simulink model "FOC_Motor_Control"  (R2020b)
settings: Solver=FixedStepAuto  StartTime=0.0  StopTime=10.0  FixedStep=Fixed_Step_Size  RelTol=1e-3
values from neighbouring files (symbols this model uses):
  Angle = 1.0    [Hall_FOC_Data.sldd]
  Angle_offset = 0.1985    [Hall_FOC_Data.sldd]
  atan_table = -1.5690511 -1.5690503 -1.5690495 -1.5690485 -1.5690477 -1.5690469 -1.569046 -1.5690452 -1.5690442 -1.5690434 -1.5690426 -1.5690417 -1.5690409 -1.5690399 -1.5690391 -1.5690383 -1.5690374 -1.5690365 -1.5690356 -1.5690348 -1.5690339 -1.569033 -1.5690322 -1.5690314 -1.5690304 -1.5690296 -1.5690287 -1.5690278 -1.5690269 -1.5690261 -1.5690252 -1.5690243 -1.5690234 -1.5690225 -1.5690217 -1.5690207 -1.569    [Hall_FOC_Data.sldd]
  Cosine_table = 1.0 0.99999529 0.99999058 0.99998587 0.99998116 0.99996704 0.99995291 0.99993885 0.99992472 0.99990118 0.99987763 0.99985409 0.9998306 0.99979764 0.99976468 0.99973178 0.99969882 0.99965644 0.99961412 0.99957174 0.99952942 0.99947762 0.99942589 0.99937415 0.99932235 0.9992612 0.99920005 0.99913889 0.99907768 0.99900717 0.99893659 0.99886602 0.99879545 0.99871546 0.99863547 0.99855554 0.99847555 0.    [Hall_FOC_Data.sldd]
  Dead_Com_Enable = 0.0    [Hall_FOC_Data.sldd]
  Dead_Time = 0.0    [Hall_FOC_Data.sldd]
  FF_Enable = 0.0    [Hall_FOC_Data.sldd]
  Flux = 0.0260812    [Hall_FOC_Data.sldd]
  FluxWeak_Enable = 0.0    [Hall_FOC_Data.sldd]
  FluxWeak_Idref_max = 0.0    [Hall_FOC_Data.sldd]
  FluxWeak_Idref_min = -200.0    [Hall_FOC_Data.sldd]
  FluxWeak_Ki = 50.0    [Hall_FOC_Data.sldd]
  FluxWeak_Kp = 1.2    [Hall_FOC_Data.sldd]
  HaLL_AngleShift = -0.25    [Hall_FOC_Data.sldd]
  HaLL_Sector1 = 5.236    [Hall_FOC_Data.sldd]
  HaLL_Sector2 = 1.0472    [Hall_FOC_Data.sldd]
  HaLL_Sector3 = 0.0    [Hall_FOC_Data.sldd]
  HaLL_Sector4 = 3.1415    [Hall_FOC_Data.sldd]
  HaLL_Sector5 = 4.1888    [Hall_FOC_Data.sldd]
  HaLL_Sector6 = 2.0944    [Hall_FOC_Data.sldd]
  HaLL_Timer_T = 1.0E-5    [Hall_FOC_Data.sldd]
  Harmonic_Com_Enable = 0.0    [Hall_FOC_Data.sldd]
  Harmonic_Id5th_Ki = 32.0    [Hall_FOC_Data.sldd]
  Harmonic_Id5th_Kp = 1.2    [Hall_FOC_Data.sldd]
  Harmonic_Id5th_Max = 60.0    [Hall_FOC_Data.sldd]
  Harmonic_Id5th_Min = -60.0    [Hall_FOC_Data.sldd]
  Harmonic_Id7th_Ki = 24.0    [Hall_FOC_Data.sldd]
  Harmonic_Id7th_Kp = 0.8    [Hall_FOC_Data.sldd]
  Harmonic_Id7th_Max = 60.0    [Hall_FOC_Data.sldd]
  Harmonic_Id7th_Min = -60.0    [Hall_FOC_Data.sldd]
  Harmonic_Iq5th_Ki = 32.0    [Hall_FOC_Data.sldd]
  Harmonic_Iq5th_Kp = 1.2    [Hall_FOC_Data.sldd]
  Harmonic_Iq5th_Max = 60.0    [Hall_FOC_Data.sldd]
  Harmonic_Iq5th_Min = -60.0    [Hall_FOC_Data.sldd]
  Harmonic_Iq7th_Ki = 24.0    [Hall_FOC_Data.sldd]
  Harmonic_Iq7th_Kp = 0.8    [Hall_FOC_Data.sldd]
  Harmonic_Iq7th_Max = 60.0    [Hall_FOC_Data.sldd]
  Harmonic_Iq7th_Min = -60.0    [Hall_FOC_Data.sldd]
  ID_Ki = 0.8    [Hall_FOC_Data.sldd]
  ID_Kp = 3.2    [Hall_FOC_Data.sldd]
  IQ_Ki = 0.32    [Hall_FOC_Data.sldd]
  IQ_Kp = 3.3    [Hall_FOC_Data.sldd]
  LADRC_b0 = 80000.0    [Hall_FOC_Data.sldd]
  LADRC_Omega_c = 80.0    [Hall_FOC_Data.sldd]
  Ld = 0.004    [Hall_FOC_Data.sldd]
  Lq = 0.0042    [Hall_FOC_Data.sldd]
  MTPA_id_table = 0.22889 0.23462678 0.23770036 0.2381243 0.23591207 0.23107713 0.2236329 0.21359272 0.20096992 0.18577772 0.16802935 0.14773798 0.12491672 0.099578641 0.071736768 0.041404068 0.0085934745 -0.026682133 -0.064409919 -0.10457709 -0.14717092 -0.1921787 -0.2395878 -0.28938559 -0.34155953 -0.39609709 -0.45298585 -0.51221335 -0.57376724 -0.63763517 -0.70380485 -0.77226412 -0.84300071 -0.91600245 -0.991257    [Hall_FOC_Data.sldd]
  MTPA_iq_table = -1.0417 -0.16083497 0.71926296 1.5985928 2.4771533 3.3549435 4.2319627 5.1082091 5.9836826 6.8583813 7.732305 8.6054525 9.4778223 10.349415 11.220228 12.090261 12.959513 13.827983 14.69567 15.562573 16.428694 17.294027 18.158575 19.022335 19.885307 20.747492 21.608887 22.469492 23.329306 24.188328 25.046556 25.903992 26.760633 27.616482 28.471533 29.325788 30.179247 31.031908 31.883772 32.734837 3    [Hall_FOC_Data.sldd]
  MTPA_Te_Max = 800.0    [Hall_FOC_Data.sldd]
  MTPA_Te_Min = 0.0    [Hall_FOC_Data.sldd]
  Over_modulation = 0.0    [Hall_FOC_Data.sldd]
  Pole_Pairs = 2.0    [Hall_FOC_Data.sldd]
  PWM_Frequency = 10000.0    [Hall_FOC_Data.sldd]
  R = 0.4    [Hall_FOC_Data.sldd]
  Sine_table = 0.0 0.0015339879 0.0030679768 0.0046019657 0.0061359555 0.0076698866 0.0092038177 0.010737749 0.012271681 0.013805497 0.015339312 0.016873131 0.018406944 0.019940587 0.021474229 0.023007872 0.024541514 0.026074925 0.027608337 0.029141748 0.03067516 0.032208283 0.033741407 0.035274528 0.036807653 0.038340431 0.039873205 0.04140598 0.042938754 0.04447113 0.046003502 0.047535874 0.049068246 0.0506001    [Hall_FOC_Data.sldd]
  Speed_Ki = 0.633    [Hall_FOC_Data.sldd]
  Speed_Kp = 0.0267    [Hall_FOC_Data.sldd]
  Speed_PI_OutputMax = 5.0    [Hall_FOC_Data.sldd]
  Speed_PI_OutputMin = -5.0    [Hall_FOC_Data.sldd]
  SpeedFilter_Fn = 0.2    [Hall_FOC_Data.sldd]
  TorqueMode = 0.0    [Hall_FOC_Data.sldd]
undefined symbols (not defined in the file or in its folder): DiscIntNeverNeededParam, inverter, magnitude, SVPWM
libraries: simulink x6, powerlib_extras x4, pid_lib x1
(part 4 of 5)

== system FOC_Motor_Control/Motor_Control/Motor_Control_Function/Angle_Speed_100us/SpeedAndAngle/ADC_IRQ/HallAngle_calibration/If Action Subsystem1 ==
  In1 : Inport
  Action Port : ActionPort  ActionPortLabel=else
  Out1 : Outport
  wires:
  In1/1 -> Out1/1

== system FOC_Motor_Control/Motor_Control/Motor_Control_Function/Angle_Speed_100us/SpeedAndAngle/ADC_IRQ/HallAngle_calibration/If Action Subsystem2 ==
  In1 : Inport
  Action Port : ActionPort  ActionPortLabel=if(u1 > 6.283185307)
  2pi : Constant  Value=2*pi  OutDataTypeStr=single
  Subtract1 : Sum  Inputs=+-  OutDataTypeStr=single
  Out1 : Outport
  wires:
  In1/1 -> Subtract1/1
  Subtract1/1 -> Out1/1
  2pi/1 -> Subtract1/2

== system FOC_Motor_Control/Motor_Control/Motor_Control_Function/Angle_Speed_100us/SpeedAndAngle/ADC_IRQ/HallAngle_calibration/If Action Subsystem3 ==
  In1 : Inport
  Action Port : ActionPort  ActionPortLabel=elseif(u1<0)
  Angle_offset : Constant  Value=2*pi  OutDataTypeStr=single
  Subtract1 : Sum
  Out1 : Outport
  wires:
  In1/1 -> Subtract1/1
  Subtract1/1 -> Out1/1
  Angle_offset/1 -> Subtract1/2

== system FOC_Motor_Control/Motor_Control/Motor_Control_Function/Control_Command_2ms/Control_Command_2ms/Speed_PI/SpeedLoop/LESO ==
  FbkSpd : Inport  OutDataTypeStr=single  PortDimensions=1
  iq : Inport  Port=2  OutDataTypeStr=single  PortDimensions=1
  Reset : Inport  Port=3
  Constant : Constant  Value=LADRC_Omega_c  OutDataTypeStr=single
  Constant1 : Constant  Value=LADRC_b0  OutDataTypeStr=single  SampleTime=-1
  Discrete-Time Integrator : DiscreteIntegrator  ExternalReset=level  SampleTime=-1  OutDataTypeStr=single  UpperSaturationLimit=6e4  LowerSaturationLimit=-6e4  ICPrevOutput=DiscIntNeverNeededParam  ICPrevScaledInput=DiscIntNeverNeededParam
  Discrete-Time Integrator1 : DiscreteIntegrator  ExternalReset=level  SampleTime=-1  OutDataTypeStr=single  LimitOutput=on  UpperSaturationLimit=2000  LowerSaturationLimit=-2000  ICPrevOutput=DiscIntNeverNeededParam  ICPrevScaledInput=DiscIntNeverNeededParam
  Gain : Gain  Gain=3  OutDataTypeStr=single
  Gain1 : Gain  Gain=2  OutDataTypeStr=single
  Product : Product  Inputs=3  OutDataTypeStr=single
  Product1 : Product  OutDataTypeStr=single
  Product2 : Product  OutDataTypeStr=single
  Sum : Sum  Inputs=|+-  OutDataTypeStr=single
  Sum1 : Sum  Inputs=+++  OutDataTypeStr=single
  omega_r_hat : Outport  OutDataTypeStr=single
  f_hat : Outport  Port=2  OutDataTypeStr=single
  wires:
  Sum/1 -> Gain1/1, Product/3
  Product/1 -> Discrete-Time Integrator/1
  Discrete-Time Integrator/1 -> [f_hat], f_hat/1
  [f_hat] -> Sum1/3
  Sum1/1 -> Discrete-Time Integrator1/1
  Discrete-Time Integrator1/1 -> omega_r_hat/1, [omega_r_hat]
  Product1/1 -> Sum1/1
  FbkSpd/1 -> Sum/1
  [omega_r_hat] -> Sum/2
  Constant/1 -> Gain/1
  Gain1/1 -> Product1/2
  Gain/1 -> Product1/1, Product/2, Product/1
  iq/1 -> Product2/1
  Constant1/1 -> Product2/2
  Product2/1 -> Sum1/2
  Reset/1 -> Discrete-Time Integrator/2, Discrete-Time Integrator1/2

== system FOC_Motor_Control/Motor_Control/Motor_Control_Function/Control_Command_2ms/Control_Command_2ms/Speed_PI/Speed_PI/Speed_Control ==
  Err : Inport
  Reset : Inport  Port=2
  Add : Sum
  Cons : Constant  Value=0  OutDataTypeStr=single
  Discrete-Time Integrator : DiscreteIntegrator  ExternalReset=level  SampleTime=-1  ICPrevOutput=DiscIntNeverNeededParam  ICPrevScaledInput=DiscIntNeverNeededParam
  Ki : Constant  Value=Speed_Ki  OutDataTypeStr=single
  Kp : Constant  Value=Speed_Kp  OutDataTypeStr=single
  Product : Product
  Product1 : Product
  Relational Operator1 : RelationalOperator  Operator===  OutDataTypeStr=boolean  RndMeth=Simplest
  Saturation : Saturate  UpperLimit=Speed_PI_OutputMax  LowerLimit=Speed_PI_OutputMin
  Scope : Scope
  Switch : Switch  Criteria=u2 > Threshold
  Unit Delay3 : UnitDelay  SampleTime=-1  HasFrameUpgradeWarning=on
  PI_Out : Outport
  wires:
  Kp/1 -> Product/1
  Err/1 -> Switch/1, Product/2
  Switch/1 -> Product1/2
  Product1/1 -> Discrete-Time Integrator/1
  Product/1 -> Add/1
  Add/1 -> Relational Operator1/1, Saturation/1
  Saturation/1 -> Relational Operator1/2, PI_Out/1
  Discrete-Time Integrator/1 -> Add/2, Scope/1
  Relational Operator1/1 -> Unit Delay3/1
  Ki/1 -> Product1/1
  Unit Delay3/1 -> Switch/2
  Cons/1 -> Switch/3
  Reset/1 -> Discrete-Time Integrator/2

== system FOC_Motor_Control/Motor_Control/Motor_Control_Function/Control_Command_2ms/Flux_weakening /Subsystem/Flux_weak/ID_Control ==
  Err : Inport
  Reset : Inport  Port=2
  Add : Sum
  Cons : Constant  Value=0  OutDataTypeStr=single
  Discrete-Time Integrator : DiscreteIntegrator  ExternalReset=level  SampleTime=-1  ICPrevOutput=DiscIntNeverNeededParam  ICPrevScaledInput=DiscIntNeverNeededParam
  Ki : Constant  Value=ki  OutDataTypeStr=single
  Kp : Constant  Value=kp  OutDataTypeStr=single
  Product : Product
  Product1 : Product
  Relational Operator1 : RelationalOperator  Operator===  OutDataTypeStr=boolean  RndMeth=Simplest
  Saturation : Saturate  UpperLimit=Id_max  LowerLimit=Id_min
  Switch : Switch  Criteria=u2 > Threshold
  Unit Delay3 : UnitDelay  SampleTime=-1  HasFrameUpgradeWarning=on
  PI_Out : Outport
  wires:
  Kp/1 -> Product/1
  Err/1 -> Switch/1, Product/2
  Switch/1 -> Product1/2
  Product1/1 -> Discrete-Time Integrator/1
  Product/1 -> Add/1
  Add/1 -> Relational Operator1/1, Saturation/1
  Saturation/1 -> Relational Operator1/2, PI_Out/1
  Cons/1 -> Switch/3
  Discrete-Time Integrator/1 -> Add/2
  Relational Operator1/1 -> Unit Delay3/1
  Ki/1 -> Product1/1
  Unit Delay3/1 -> Switch/2
  Reset/1 -> Discrete-Time Integrator/2

== system FOC_Motor_Control/Motor_Control/Motor_Control_Function/Control_Command_2ms/Flux_weakening /Subsystem/Flux_weak/Normal ==
  Bus_voltage : Inport
  Action Port : ActionPort  ActionPortLabel=elseif(u1==0)
  Gain : Gain  Gain=1/sqrt(3)
  Out1 : Outport
  wires:
  Bus_voltage/1 -> Gain/1
  Gain/1 -> Out1/1

== system FOC_Motor_Control/Motor_Control/Motor_Control_Function/Control_Command_2ms/Flux_weakening /Subsystem/Flux_weak/Over_M ==
  Bus_voltage : Inport
  Action Port : ActionPort  ActionPortLabel=if(u1==1)
  Gain : Gain  Gain=2/3
  Out1 : Outport
  wires:
  Bus_voltage/1 -> Gain/1
  Gain/1 -> Out1/1

== system FOC_Motor_Control/Motor_Control/Motor_Control_Function/FOC_Control_100us/FOC/DT_Compensation/DT_Compensation/IsTheta_Cal ==
  Id : Inport
  Iq : Inport  Port=2
  d_theta : Inport  Port=3
  Add1 : Sum
  Angle_calibration : Subsystem
      settings: RTWSystemCode=Nonreusable function  RTWFcnNameOpts=Use subsystem name
  LPF : Subsystem
  LPF1 : Subsystem
  Scope2 : Scope  NumInputPorts=2
  Scope3 : Scope  NumInputPorts=2
  atan : Subsystem
  IsTheta : Outport
  wires:
  d_theta/1 -> Add1/2
  Angle_calibration/1(Angle_output) -> IsTheta/1
  Iq/1 -> LPF/1(u), Scope2/1
  Id/1 -> LPF1/1(u), Scope3/1
  LPF1/1(y) -> [B_Id], Scope3/2
  LPF/1(y) -> Scope2/2, [A_Iq]
  Add1/1 -> Angle_calibration/1(Angle_input)  "Itheta2"
  [A_Iq] -> atan/1(Id)
  [B_Id] -> atan/2(Iq)
  atan/1(Out1) -> Add1/1

== system FOC_Motor_Control/Motor_Control/Motor_Control_Function/FOC_Control_100us/FOC/DT_Compensation/DT_Compensation/Subsystem ==
  Err_Voltage : Inport
  Istheta : Inport  Port=2
  If1 : If  IfExpression=(u1 >5.75958)|(u1<=0.523598)  ElseIfExpressions=(u1 >0.523598)&(u1<=1.570796),(u1 >1.570796)&(u1<=2.617993),(u1 >2.617993)&(u1<=3.665191),(u1 >3.665191)&(u1<=4.7123889),(u1 >4.7123889)&(u1<=5.75958)  ShowElse=off
  Merge : Merge  Inputs=6
  Subsystem : Subsystem
  Subsystem1 : Subsystem
  Subsystem2 : Subsystem
  Subsystem3 : Subsystem
  Subsystem4 : Subsystem
  Subsystem5 : Subsystem
  Uabcc : Outport
  wires:
  Istheta/1 -> If1/1
  If1/1 -> Subsystem/Action
  If1/2 -> Subsystem1/Action
  If1/3 -> Subsystem2/Action
  If1/4 -> Subsystem3/Action
  If1/5 -> Subsystem4/Action
  If1/6 -> Subsystem5/Action
  Err_Voltage/1 -> Subsystem5/1(Voltage), Subsystem3/1(Voltage), Subsystem2/1(Voltage), Subsystem/1(Voltage), Subsystem1/1(Voltage), Subsystem4/1(Voltage)
  Merge/1 -> Uabcc/1
  Subsystem/1(Out1) -> Merge/1
  Subsystem1/1(Out1) -> Merge/2
  Subsystem2/1(Out1) -> Merge/3
  Subsystem3/1(Out1) -> Merge/4
  Subsystem4/1(Out1) -> Merge/5
  Subsystem5/1(Out1) -> Merge/6

== system FOC_Motor_Control/Motor_Control/Motor_Control_Function/FOC_Control_100us/FOC/DT_Compensation/DT_Compensation/Uabc_alphabeta ==
  Uabc : Inport
  Fcn : Fcn  Expr=(2/3)*(u(1)-0.5*u(2)-0.5*u(3))
  Fcn1 : Fcn  Expr=sqrt(1/3)*(u(2)-u(3))
  Ualpha : Outport
  Ubeta : Outport  Port=2
  wires:
  Fcn/1 -> Ualpha/1
  Fcn1/1 -> Ubeta/1
  Uabc/1 -> Fcn1/1, Fcn/1

== system FOC_Motor_Control/Motor_Control/Motor_Control_Function/FOC_Control_100us/FOC/D_Current_PI/ID_Control/Normal ==
  Bus_voltage : Inport
  Action Port : ActionPort  ActionPortLabel=elseif(u1==0)
  Gain : Gain  Gain=1/sqrt(3)
  Gain1 : Gain  Gain=-1/sqrt(3)
  Out1 : Outport
  Out2 : Outport  Port=2
  wires:
  Bus_voltage/1 -> Gain1/1, Gain/1
  Gain/1 -> Out1/1
  Gain1/1 -> Out2/1

== system FOC_Motor_Control/Motor_Control/Motor_Control_Function/FOC_Control_100us/FOC/D_Current_PI/ID_Control/Over_M ==
  Bus_voltage : Inport
  Action Port : ActionPort  ActionPortLabel=if(u1==1)
  Gain : Gain  Gain=2/3
  Gain1 : Gain  Gain=-2/3
  Out1 : Outport
  Out2 : Outport  Port=2
  wires:
  Bus_voltage/1 -> Gain1/1, Gain/1
  Gain/1 -> Out1/1
  Gain1/1 -> Out2/1

== system FOC_Motor_Control/Motor_Control/Motor_Control_Function/FOC_Control_100us/FOC/Har_Compensation/Har_Compensation/Idq5 ==
  Ialpha : Inport
  Ibeta : Inport  Port=2
  Cos_theta : Inport  Port=3
  Sin_theta : Inport  Port=4
  LPF : Subsystem
  LPF2 : Subsystem
  Mux : Mux  Inputs=2
  Park1 : Subsystem
  Scope : Scope  NumInputPorts=2
  Idq5 : Outport  VectorParamsAs1DForOutWhenUnconnected=off
  wires:
  Park1/1(Id5) -> Mux/1
  Park1/2(Iq5) -> Mux/2
  Mux/1 -> Scope/1, LPF/1(u)
  Cos_theta/1 -> Park1/3(Cos_theta)
  Sin_theta/1 -> Park1/4(Sin_theta)
  Ialpha/1 -> Park1/1(Ialf)
  Ibeta/1 -> Park1/2(Ibelt)
  LPF/1(y) -> LPF2/1(u)
  LPF2/1(y) -> Scope/2, Idq5/1

== system FOC_Motor_Control/Motor_Control/Motor_Control_Function/FOC_Control_100us/FOC/Har_Compensation/Har_Compensation/Idq7 ==
  Ialpha : Inport
  Ibeta : Inport  Port=2
  Cos_theta : Inport  Port=3
  Sin_theta : Inport  Port=4
  LPF : Subsystem
  LPF2 : Subsystem
  Mux : Mux  Inputs=2
  Park1 : Subsystem
  Idq7 : Outport  VectorParamsAs1DForOutWhenUnconnected=off
  wires:
  Park1/2(Iq7) -> Mux/2
  Ibeta/1 -> Park1/2(Ibelt)
  Ialpha/1 -> Park1/1(Ialf)
  Park1/1(Id7) -> Mux/1
  Mux/1 -> LPF/1(u)
  Sin_theta/1 -> Park1/4(Sin_theta)
  Cos_theta/1 -> Park1/3(Cos_theta)
  LPF/1(y) -> LPF2/1(u)
  LPF2/1(y) -> Idq7/1

== system FOC_Motor_Control/Motor_Control/Motor_Control_Function/FOC_Control_100us/FOC/Har_Compensation/Har_Compensation/Sine_Cosine1 ==
  note: Sine Cosine Coefficients
  P : Inport
  Cosine : Lookup_n-D  NumberOfTableDimensions=1  LookupTableObject=''  BreakpointsForDimension1=[0:2*pi/4095:2*pi]  BreakpointsForDimension1FirstPoint=10  BreakpointsForDimension2FirstPoint=10  BreakpointsForDimension1Spacing=12  BreakpointsForDimension2Spacing=12  IndexSearchMethod=Evenly spaced points  Table=Cosine_table  InterpMethod=Flat  DiagnosticForOutOfRangeInput=Error  InternalRulePriority=Speed  RndMeth=Simplest  InputSameDT=on
  Saturation : Saturate  UpperLimit=2*pi-0.0001  LowerLimit=0+0.0001
  Scope : Scope  NumInputPorts=2
  Sine : Lookup_n-D  NumberOfTableDimensions=1  LookupTableObject=''  BreakpointsForDimension1=[0:2*pi/4095:2*pi]  BreakpointsForDimension1FirstPoint=10  BreakpointsForDimension2FirstPoint=10  BreakpointsForDimension1Spacing=12  BreakpointsForDimension2Spacing=12  IndexSearchMethod=Evenly spaced points  Table=Sine_table  InterpMethod=Flat  DiagnosticForOutOfRangeInput=Error  InternalRulePriority=Speed  RndMeth=Simplest  InputSameDT=on
  Cos : Outport  VectorParamsAs1DForOutWhenUnconnected=off
  Sin : Outport  Port=2  VectorParamsAs1DForOutWhenUnconnected=off
  wires:
  P/1 -> Saturation/1  "position"
  Sine/1 -> Scope/1, Sin/1
  Cosine/1 -> Scope/2, Cos/1
  Saturation/1 -> Cosine/1, Sine/1

== system FOC_Motor_Control/Motor_Control/Motor_Control_Function/FOC_Control_100us/FOC/Har_Compensation/Har_Compensation/Sine_Cosine2 ==
  note: Sine Cosine Coefficients
  P : Inport
  Cosine : Lookup_n-D  NumberOfTableDimensions=1  LookupTableObject=''  BreakpointsForDimension1=[0:2*pi/4095:2*pi]  BreakpointsForDimension1FirstPoint=10  BreakpointsForDimension2FirstPoint=10  BreakpointsForDimension1Spacing=12  BreakpointsForDimension2Spacing=12  IndexSearchMethod=Evenly spaced points  Table=Cosine_table  InterpMethod=Flat  DiagnosticForOutOfRangeInput=Error  InternalRulePriority=Speed  RndMeth=Simplest  InputSameDT=on
  Saturation : Saturate  UpperLimit=2*pi-0.0001  LowerLimit=0+0.0001
  Scope : Scope  NumInputPorts=2
  Sine : Lookup_n-D  NumberOfTableDimensions=1  LookupTableObject=''  BreakpointsForDimension1=[0:2*pi/4095:2*pi]  BreakpointsForDimension1FirstPoint=10  BreakpointsForDimension2FirstPoint=10  BreakpointsForDimension1Spacing=12  BreakpointsForDimension2Spacing=12  IndexSearchMethod=Evenly spaced points  Table=Sine_table  InterpMethod=Flat  DiagnosticForOutOfRangeInput=Error  InternalRulePriority=Speed  RndMeth=Simplest  InputSameDT=on
  Cos : Outport  VectorParamsAs1DForOutWhenUnconnected=off
  Sin : Outport  Port=2  VectorParamsAs1DForOutWhenUnconnected=off
  wires:
  P/1 -> Saturation/1  "position"
  Sine/1 -> Scope/1, Sin/1
  Cosine/1 -> Scope/2, Cos/1
  Saturation/1 -> Cosine/1, Sine/1

== system FOC_Motor_Control/Motor_Control/Motor_Control_Function/FOC_Control_100us/FOC/Har_Compensation/Har_Compensation/Switch_2pi ==
  Input : Inport
  Data Type Conversion : DataTypeConversion  OutDataTypeStr=int32
  Divide : Product  Inputs=*/
  Divide1 : Product  Inputs=**
  Subtract : Sum  Inputs=-+
  Te2 : Constant  Value=2*pi  OutDataTypeStr=single
  Te3 : Constant  Value=2*pi  OutDataTypeStr=single
  output : Outport
  wires:
  Te3/1 -> Divide1/2
  Data Type Conversion/1 -> Divide1/1
  Divide/1 -> Data Type Conversion/1
  Divide1/1 -> Subtract/1
  Te2/1 -> Divide/2
  Subtract/1 -> output/1
  Input/1 -> Subtract/2, Divide/1

== system FOC_Motor_Control/Motor_Control/Motor_Control_Function/FOC_Control_100us/FOC/Har_Compensation/Har_Compensation/Switch_2pi1 ==
  Input : Inport
  Data Type Conversion : DataTypeConversion  OutDataTypeStr=int32
  Divide : Product  Inputs=*/
  Divide1 : Product  Inputs=**
  Subtract : Sum  Inputs=-+
  Te2 : Constant  Value=2*pi  OutDataTypeStr=single
  Te3 : Constant  Value=2*pi  OutDataTypeStr=single
  output : Outport
  wires:
  Te3/1 -> Divide1/2
  Data Type Conversion/1 -> Divide1/1
  Divide/1 -> Data Type Conversion/1
  Divide1/1 -> Subtract/1
  Te2/1 -> Divide/2
  Subtract/1 -> output/1
  Input/1 -> Subtract/2, Divide/1

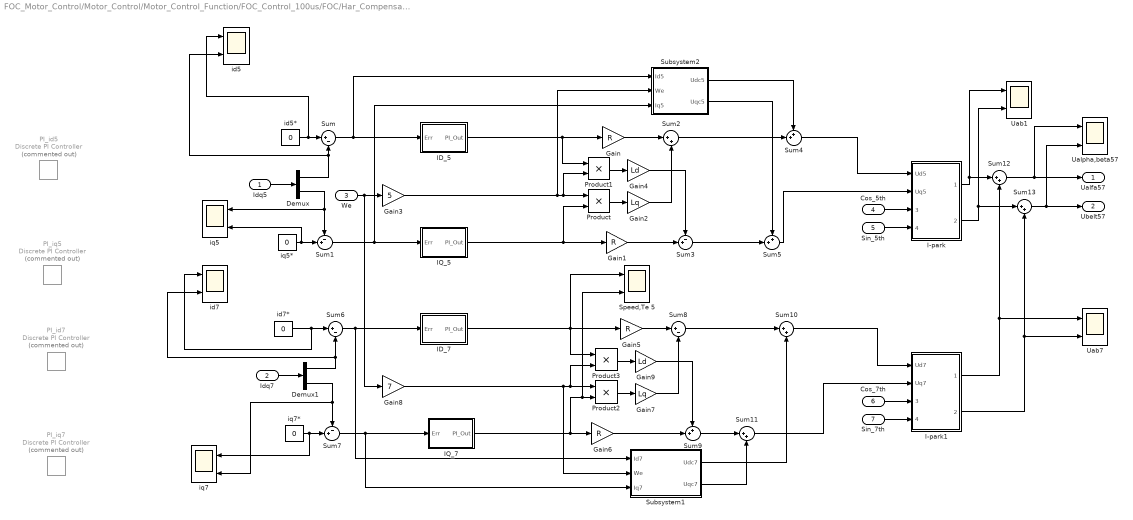
== system FOC_Motor_Control/Motor_Control/Motor_Control_Function/FOC_Control_100us/FOC/Har_Compensation/Har_Compensation/idq57_Controller ==
  Idq5 : Inport
  Idq7 : Inport  Port=2
  We : Inport  Port=3
  Cos_5th : Inport  Port=4
  Sin_5th : Inport  Port=5
  Cos_7th : Inport  Port=6
  Sin_7th : Inport  Port=7
  Demux : Demux  Outputs=2
  Demux1 : Demux  Outputs=2
  Gain{,1,5..6} (4 alike) : Gain  Gain=R
  Gain2 : Gain  Gain=Lq
  Gain3 : Gain  Gain=5
  Gain4 : Gain  Gain=Ld
  Gain7 : Gain  Gain=Lq
  Gain8 : Gain  Gain=7
  Gain9 : Gain  Gain=Ld
  I-park : Subsystem
  I-park1 : Subsystem
  ID_5 : Subsystem
  ID_7 : Subsystem
  IQ_5 : Subsystem
  IQ_7 : Subsystem
  PI_id5 : powerlib_extras/Discrete  Control Blocks/Discrete PI Controller  Commented=on  Kp=Harmonic_Id5th_Kp  Ki=Harmonic_Id5th_Ki  Par_Limits=[60 -60]  Init=0  Ts=-1
  PI_id7 : powerlib_extras/Discrete  Control Blocks/Discrete PI Controller  Commented=on  Kp=Harmonic_Id7th_Kp  Ki=Harmonic_Id7th_Ki  Par_Limits=[60 -60]  Init=0  Ts=-1
  PI_iq5 : powerlib_extras/Discrete  Control Blocks/Discrete PI Controller  Commented=on  Kp=Harmonic_Iq5th_Kp  Ki=Harmonic_Iq5th_Ki  Par_Limits=[60 -60]  Init=0  Ts=-1
  PI_iq7 : powerlib_extras/Discrete  Control Blocks/Discrete PI Controller  Commented=on  Kp=Harmonic_Iq7th_Kp  Ki=Harmonic_Iq7th_Ki  Par_Limits=[60 -60]  Init=0  Ts=-1
  Product{,1..3} (4 alike) : Product
  Speed,Te 5 : Scope  NumInputPorts=2
  Subsystem1 : Subsystem
  Subsystem2 : Subsystem
  Sum : Sum  Inputs=|+-
  Sum1 : Sum  Inputs=-+|
  Sum{2,10..13} (5 alike) : Sum  Inputs=|++
  Sum3 : Sum  Inputs=-+|
  Sum4 : Sum  Inputs=++|
  Sum5 : Sum  Inputs=++|
  Sum6 : Sum  Inputs=|+-
  Sum7 : Sum  Inputs=-+|
  Sum8 : Sum  Inputs=|+-
  Sum9 : Sum  Inputs=++|
  Uab1 : Scope  NumInputPorts=2
  Uab7 : Scope  NumInputPorts=2
  Ualpha,beta57 : Scope  NumInputPorts=2
  id5 : Scope  NumInputPorts=2
  id5* : Constant  Value=0  OutDataTypeStr=single
  id7 : Scope  NumInputPorts=2
  id7* : Constant  Value=0  OutDataTypeStr=single
  iq5 : Scope  NumInputPorts=2
  iq5* : Constant  Value=0  OutDataTypeStr=single
  iq7 : Scope  NumInputPorts=2
  iq7* : Constant  Value=0  OutDataTypeStr=single
  Ualfa57 : Outport  VectorParamsAs1DForOutWhenUnconnected=off
  Ubelt57 : Outport  Port=2  VectorParamsAs1DForOutWhenUnconnected=off
  wires:
  Idq5/1 -> Demux/1
  id5*/1 -> id5/1, Sum/1
  Demux/1 -> id5/2, Sum/2
  Demux/2 -> Sum1/1, iq5/1
  Sum/1 -> ID_5/1(Err), Subsystem2/1(Id5)
  Sum1/1 -> IQ_5/1(Err), Subsystem2/3(Iq5)
  ID_5/1(PI_Out) -> Gain/1, Product1/1
  IQ_5/1(PI_Out) -> Product/2, Gain1/1
  Gain/1 -> Sum2/1
  Product/1 -> Gain2/1
  Gain2/1 -> Sum2/2
  Gain3/1 -> Subsystem2/2(We), Product/1, Product1/2
  Gain1/1 -> Sum3/2
  Product1/1 -> Gain4/1
  Gain4/1 -> Sum3/1
  Gain9/1 -> Sum9/1
  Product3/1 -> Gain9/1
  Gain6/1 -> Sum9/2
  Gain8/1 -> Subsystem1/2(We), Product3/2, Product2/1
  Gain7/1 -> Sum8/2
  Product2/1 -> Gain7/1
  We/1 -> Gain8/1, Gain3/1
  Gain5/1 -> Sum8/1
  IQ_7/1(PI_Out) -> Gain6/1, Speed,Te 5/2, Product2/2
  ID_7/1(PI_Out) -> Product3/1, Speed,Te 5/1, Gain5/1
  Sum7/1 -> IQ_7/1(Err), Subsystem1/3(Iq7)
  Sum6/1 -> ID_7/1(Err), Subsystem1/1(Id7)
  iq7*/1 -> iq7/1, Sum7/2
  id7*/1 -> id7/1, Sum6/1
  Idq7/1 -> Demux1/1
  I-park/1(Ualfa5) -> Uab1/1, Sum12/1
  I-park/2(Ubelt5) -> Uab1/2, Sum13/1
  Sum13/1 -> Ualpha,beta57/2, Ubelt57/1
  Demux1/1 -> Sum6/2, id7/2
  Sum12/1 -> Ualpha,beta57/1, Ualfa57/1
  Sum2/1 -> Sum4/2
  Sum4/1 -> I-park/1(Ud5)
  Sum3/1 -> Sum5/2
  Sum5/1 -> I-park/2(Uq5)
  Sum8/1 -> Sum10/1
  Sum9/1 -> Sum11/1
  Sum10/1 -> I-park1/1(Ud7)
  Sum11/1 -> I-park1/2(Uq7)
  iq5*/1 -> iq5/2, Sum1/2
  I-park1/2(Ubelt7) -> Uab7/2, Sum13/2
  Demux1/2 -> iq7/2, Sum7/1
  Subsystem2/1(Udc5) -> Sum4/1
  Subsystem2/2(Uqc5) -> Sum5/1
  Subsystem1/1(Udc7) -> Sum10/2
  Subsystem1/2(Uqc7) -> Sum11/2
  I-park1/1(Ualfa7) -> Sum12/2, Uab7/1
  Cos_5th/1 -> I-park/3(Cos_theta)
  Sin_5th/1 -> I-park/4(Sin_theta)
  Cos_7th/1 -> I-park1/3(Cos_theta)
  Sin_7th/1 -> I-park1/4(Sin_theta)

== system FOC_Motor_Control/Motor_Control/Motor_Control_Function/FOC_Control_100us/FOC/Q_Current_PI/IQ_Control/Normal ==
  Bus_voltage : Inport
  Action Port : ActionPort  ActionPortLabel=elseif(u1==0)
  Gain : Gain  Gain=1/sqrt(3)
  Gain1 : Gain  Gain=-1/sqrt(3)
  Out1 : Outport
  Out2 : Outport  Port=2
  wires:
  Bus_voltage/1 -> Gain1/1, Gain/1
  Gain/1 -> Out1/1
  Gain1/1 -> Out2/1

== system FOC_Motor_Control/Motor_Control/Motor_Control_Function/FOC_Control_100us/FOC/Q_Current_PI/IQ_Control/Over_M ==
  Bus_voltage : Inport
  Action Port : ActionPort  ActionPortLabel=if(u1==1)
  Gain : Gain  Gain=2/3
  Gain1 : Gain  Gain=-2/3
  Out1 : Outport
  Out2 : Outport  Port=2
  wires:
  Bus_voltage/1 -> Gain1/1, Gain/1
  Gain/1 -> Out1/1
  Gain1/1 -> Out2/1

== system FOC_Motor_Control/Motor_Control/Motor_Control_Function/FOC_Control_100us/FOC/DT_Compensation/DT_Compensation/IsTheta_Cal/Angle_calibration ==
  Angle_input : Inport
  If Action Subsystem1 : Subsystem  TreatAsAtomicUnit=on
  If Action Subsystem2 : Subsystem  TreatAsAtomicUnit=on
  If1 : If  IfExpression=u1 > 6.283185307
  Merge1 : Merge
  Angle_output : Outport
  wires:
  Merge1/1 -> Angle_output/1
  If1/1 -> If Action Subsystem2/Action
  If1/2 -> If Action Subsystem1/Action
  If Action Subsystem2/1(Out1) -> Merge1/1
  Angle_input/1 -> If Action Subsystem1/1(Angle_input), If Action Subsystem2/1(In1), If1/1
  If Action Subsystem1/1(Out1) -> Merge1/2

== system FOC_Motor_Control/Motor_Control/Motor_Control_Function/FOC_Control_100us/FOC/DT_Compensation/DT_Compensation/IsTheta_Cal/LPF ==
  u : Inport
  Add : Sum  Inputs=+-
  Add1 : Sum
  Constant1 : Constant  Value=0.005  OutDataTypeStr=single
  Divide1 : Product  Inputs=**
  Unit Delay : UnitDelay  SampleTime=-1  HasFrameUpgradeWarning=on
  y : Outport
  wires:
  Constant1/1 -> Divide1/1
  u/1 -> Add/1
  Add/1 -> Divide1/2
  Divide1/1 -> Add1/1
  Unit Delay/1 -> Add/2, Add1/2
  Add1/1 -> Unit Delay/1, y/1

== system FOC_Motor_Control/Motor_Control/Motor_Control_Function/FOC_Control_100us/FOC/DT_Compensation/DT_Compensation/IsTheta_Cal/LPF1 ==
  u : Inport
  Add : Sum  Inputs=+-
  Add1 : Sum
  Constant1 : Constant  Value=0.005  OutDataTypeStr=single
  Divide1 : Product  Inputs=**
  Unit Delay : UnitDelay  SampleTime=-1  HasFrameUpgradeWarning=on
  y : Outport
  wires:
  Constant1/1 -> Divide1/1
  u/1 -> Add/1
  Add/1 -> Divide1/2
  Divide1/1 -> Add1/1
  Unit Delay/1 -> Add/2, Add1/2
  Add1/1 -> Unit Delay/1, y/1

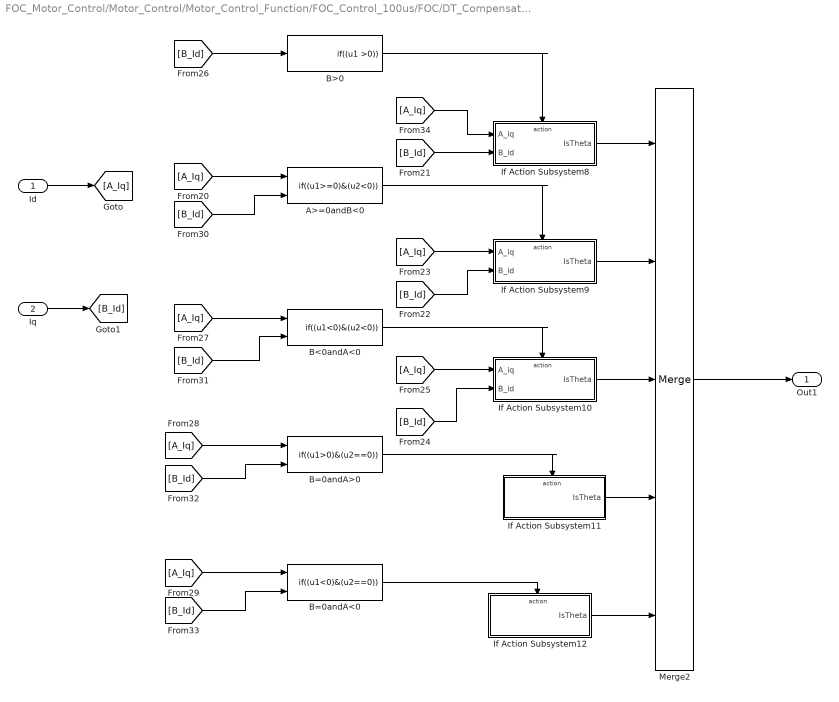
== system FOC_Motor_Control/Motor_Control/Motor_Control_Function/FOC_Control_100us/FOC/DT_Compensation/DT_Compensation/IsTheta_Cal/atan ==
  Id : Inport
  Iq : Inport  Port=2
  A>=0andB<0 : If  NumInputs=2  IfExpression=(u1>=0)&(u2<0)  ShowElse=off
  B<0andA<0 : If  NumInputs=2  IfExpression=(u1<0)&(u2<0)  ShowElse=off
  B=0andA<0 : If  NumInputs=2  IfExpression=(u1<0)&(u2==0)  ShowElse=off
  B=0andA>0 : If  NumInputs=2  IfExpression=(u1>0)&(u2==0)  ShowElse=off
  B>0 : If  IfExpression=(u1 >0)  ShowElse=off
  If Action Subsystem10 : Subsystem  TreatAsAtomicUnit=on
  If Action Subsystem11 : Subsystem  TreatAsAtomicUnit=on
  If Action Subsystem12 : Subsystem  TreatAsAtomicUnit=on
  If Action Subsystem8 : Subsystem  TreatAsAtomicUnit=on
  If Action Subsystem9 : Subsystem  TreatAsAtomicUnit=on
  Merge2 : Merge  Inputs=5
  Out1 : Outport
  wires:
  B<0andA<0/1 -> If Action Subsystem10/Action
  [A_Iq] -> If Action Subsystem10/1(A_iq)
  B=0andA<0/1 -> If Action Subsystem12/Action
  B=0andA>0/1 -> If Action Subsystem11/Action
  [A_Iq] -> If Action Subsystem8/1(A_iq)
  [B_Id] -> B>0/1
  A>=0andB<0/1 -> If Action Subsystem9/Action
  If Action Subsystem11/1(IsTheta) -> Merge2/4
  If Action Subsystem9/1(IsTheta) -> Merge2/2
  [B_Id] -> If Action Subsystem9/2(B_id)
  B>0/1 -> If Action Subsystem8/Action
  [A_Iq] -> If Action Subsystem9/1(A_iq)
  If Action Subsystem8/1(IsTheta) -> Merge2/1
  [B_Id] -> B<0andA<0/2
  [A_Iq] -> A>=0andB<0/1
  [B_Id] -> B=0andA<0/2
  [B_Id] -> A>=0andB<0/2
  [A_Iq] -> B=0andA<0/1
  [A_Iq] -> B=0andA>0/1
  [A_Iq] -> B<0andA<0/1
  [B_Id] -> B=0andA>0/2
  If Action Subsystem12/1(IsTheta) -> Merge2/5
  If Action Subsystem10/1(IsTheta) -> Merge2/3
  Merge2/1 -> Out1/1
  [B_Id] -> If Action Subsystem8/2(B_id)
  [B_Id] -> If Action Subsystem10/2(B_id)
  Id/1 -> [A_Iq]
  Iq/1 -> [B_Id]

== system FOC_Motor_Control/Motor_Control/Motor_Control_Function/FOC_Control_100us/FOC/DT_Compensation/DT_Compensation/Subsystem/Subsystem ==
  Voltage : Inport
  Action Port : ActionPort  ActionPortLabel=if((u1 >5.75958)|(u1<=0.523598))
  Gain : Gain
  Gain1 : Gain  Gain=-1
  Gain2 : Gain  Gain=-1
  Mux1 : Mux  Inputs=3
  Out1 : Outport
  wires:
  Gain/1 -> Mux1/1
  Gain1/1 -> Mux1/2
  Voltage/1 -> Gain2/1, Gain1/1, Gain/1
  Gain2/1 -> Mux1/3
  Mux1/1 -> Out1/1

== system FOC_Motor_Control/Motor_Control/Motor_Control_Function/FOC_Control_100us/FOC/DT_Compensation/DT_Compensation/Subsystem/Subsystem1 ==
  Voltage : Inport
  Action Port : ActionPort  ActionPortLabel=elseif((u1 >0.523598)&(u1<=1.570796))
  Gain : Gain
  Gain1 : Gain
  Gain2 : Gain  Gain=-1
  Mux1 : Mux  Inputs=3
  Out1 : Outport
  wires:
  Mux1/1 -> Out1/1
  Voltage/1 -> Gain2/1, Gain1/1, Gain/1
  Gain/1 -> Mux1/1
  Gain1/1 -> Mux1/2
  Gain2/1 -> Mux1/3
